simulink model "analog_ext1"  (Simulink 7.6)
settings: Solver=FixedStepDiscrete  StartTime=0.0  StopTime=10.0  FixedStep=1  RelTol=1e-3
libraries: simulink x5
settings Model: Creator=jordan  LastModifiedBy=jordan
settings DataIOCC: LimitDataPoints=off  SaveOutput=off  SignalLogging=off  DSMLogging=off  SaveTime=off
settings OptimizationCC: BlockReduction=off  ConditionallyExecuteInputs=off

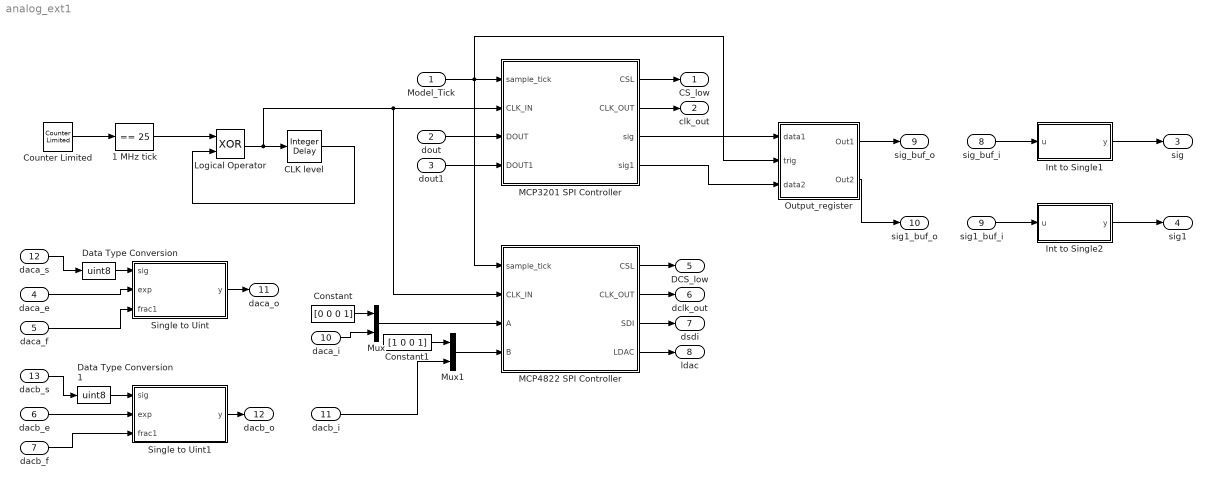
== system analog_ext1 ==
  Model_Tick : Inport  OutDataTypeStr=boolean
  dout : Inport  Port=2  OutDataTypeStr=boolean
  dout1 : Inport  Port=3  OutDataTypeStr=boolean
  daca_e : Inport  Port=4  OutDataTypeStr=uint8
  daca_f : Inport  Port=5  OutDataTypeStr=fixdt(0,24,0)
  dacb_e : Inport  Port=6  OutDataTypeStr=uint8
  dacb_f : Inport  Port=7  OutDataTypeStr=fixdt(0,24,0)
  sig_buf_i : Inport  Port=8  OutDataTypeStr=fixdt(0,12,0)
  sig1_buf_i : Inport  Port=9  OutDataTypeStr=fixdt(0,12,0)
  daca_i : Inport  Port=10  OutDataTypeStr=boolean  PortDimensions=12
  dacb_i : Inport  Port=11  OutDataTypeStr=boolean  PortDimensions=12
  daca_s : Inport  Port=12  OutDataTypeStr=boolean
  dacb_s : Inport  Port=13  OutDataTypeStr=boolean
  1 MHz tick : simulink/Logic and Bit Operations/Compare To Constant  SystemSampleTime=-1  relop===  const=25  LogicOutDataTypeMode=boolean
  CLK level : simulink/Discrete/Integer Delay  NumDelays=1  vinit=0.0  samptime=-1
  Constant : Constant  Value=[0 0 0 1]  OutDataTypeStr=boolean
  Constant1 : Constant  Value=[1 0 0 1]  OutDataTypeStr=boolean
  Counter Limited : simulink/Sources/Counter Limited  SystemSampleTime=-1  uplimit=50  tsamp=-1
  Data Type Conversion : DataTypeConversion  OutDataTypeStr=uint8
  Data Type Conversion1 : DataTypeConversion  OutDataTypeStr=uint8
  Int to Single1 : Stateflow chart  TreatAsAtomicUnit=on
  Int to Single2 : Stateflow chart  TreatAsAtomicUnit=on
  Logical Operator : Logic  Operator=XOR  AllPortsSameDT=off  OutDataTypeStr=boolean
  MCP3201 SPI Controller : Stateflow chart  TreatAsAtomicUnit=on
  MCP4822 SPI Controller : Stateflow chart  TreatAsAtomicUnit=on
  Mux : Mux  Inputs=2
  Mux1 : Mux  Inputs=2
  Output_register : Subsystem
  Single to Uint : Stateflow chart  TreatAsAtomicUnit=on
  Single to Uint1 : Stateflow chart  TreatAsAtomicUnit=on
  CS_low : Outport  OutDataTypeStr=boolean
  clk_out : Outport  Port=2  OutDataTypeStr=boolean
  sig : Outport  Port=3  OutDataTypeStr=uint32  PortDimensions=1
  sig1 : Outport  Port=4  OutDataTypeStr=uint32  PortDimensions=1
  DCS_low : Outport  Port=5  OutDataTypeStr=boolean
  dclk_out : Outport  Port=6  OutDataTypeStr=boolean
  dsdi : Outport  Port=7  OutDataTypeStr=boolean
  ldac : Outport  Port=8  OutDataTypeStr=boolean
  sig_buf_o : Outport  Port=9  OutDataTypeStr=boolean  PortDimensions=12
  sig1_buf_o : Outport  Port=10  OutDataTypeStr=boolean  PortDimensions=12
  daca_o : Outport  Port=11  OutDataTypeStr=fixdt(0,12,0)
  dacb_o : Outport  Port=12  OutDataTypeStr=fixdt(0,12,0)
  wires:
  Counter Limited/1 -> 1 MHz tick/1
  1 MHz tick/1 -> Logical Operator/1
  Logical Operator/1 -> CLK level/1, MCP3201 SPI Controller/2(CLK_IN), MCP4822 SPI Controller/2(CLK_IN)
  CLK level/1 -> Logical Operator/2
  Model_Tick/1 -> MCP3201 SPI Controller/1(sample_tick), MCP4822 SPI Controller/1(sample_tick), Output_register/2(trig)
  MCP3201 SPI Controller/1(CSL) -> CS_low/1
  MCP3201 SPI Controller/2(CLK_OUT) -> clk_out/1
  MCP3201 SPI Controller/3(sig) -> Output_register/1(data1)
  dout/1 -> MCP3201 SPI Controller/3(DOUT)
  MCP3201 SPI Controller/4(sig1) -> Output_register/3(data2)
  dout1/1 -> MCP3201 SPI Controller/4(DOUT1)
  Mux1/1 -> MCP4822 SPI Controller/4(B)
  Constant/1 -> Mux/1
  Mux/1 -> MCP4822 SPI Controller/3(A)
  Constant1/1 -> Mux1/1
  MCP4822 SPI Controller/1(CSL) -> DCS_low/1
  MCP4822 SPI Controller/2(CLK_OUT) -> dclk_out/1
  MCP4822 SPI Controller/3(SDI) -> dsdi/1
  MCP4822 SPI Controller/4(LDAC) -> ldac/1
  Output_register/1(Out1) -> sig_buf_o/1
  Output_register/2(Out2) -> sig1_buf_o/1
  Int to Single1/1(y) -> sig/1
  Int to Single2/1(y) -> sig1/1
  Single to Uint/1(y) -> daca_o/1
  Single to Uint1/1(y) -> dacb_o/1
  daca_s/1 -> Data Type Conversion/1
  daca_e/1 -> Single to Uint/2(exp)
  daca_f/1 -> Single to Uint/3(frac1)
  dacb_e/1 -> Single to Uint1/2(exp)
  dacb_f/1 -> Single to Uint1/3(frac1)
  sig_buf_i/1 -> Int to Single1/1(u)
  sig1_buf_i/1 -> Int to Single2/1(u)
  daca_i/1 -> Mux/2
  dacb_i/1 -> Mux1/2
  dacb_s/1 -> Data Type Conversion1/1
  Data Type Conversion/1 -> Single to Uint/1(sig)
  Data Type Conversion1/1 -> Single to Uint1/1(sig)

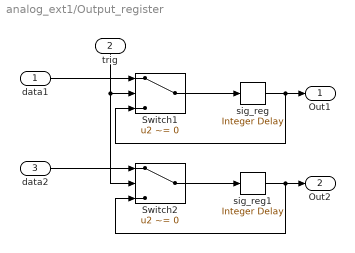
== system analog_ext1/Output_register ==
  data1 : Inport
  trig : Inport  Port=2
  data2 : Inport  Port=3
  Switch1 : Switch  Criteria=u2 ~= 0
  Switch2 : Switch  Criteria=u2 ~= 0
  sig_reg : simulink/Discrete/Integer Delay  NumDelays=1  vinit=0.0  samptime=-1
  sig_reg1 : simulink/Discrete/Integer Delay  NumDelays=1  vinit=0.0  samptime=-1
  Out1 : Outport
  Out2 : Outport  Port=2
  wires:
  Switch1/1 -> sig_reg/1
  sig_reg/1 -> Switch1/3, Out1/1
  Switch2/1 -> sig_reg1/1
  sig_reg1/1 -> Switch2/3, Out2/1
  trig/1 -> Switch2/2, Switch1/2
  data1/1 -> Switch1/1
  data2/1 -> Switch2/1

== stateflow chart MCP3201 SPI Controller ==
  settings: executeAtInitialization=1
  state Wait_Request
  state Get_Sample
  state Wait_CLK_0
  state Get_Sample1
  state Get_Sample2
  state Get_Sample3
  state Receive_Data
  state Receive_Data1
  state Receive_Data2
  state Get_Sample4
  state Get_Sample5
  (default) -> Wait_Request : {CSL=1;
      | CLK_OUT=0;}
  Wait_Request -> Wait_CLK_0 : [sample_tick]
  Wait_CLK_0 -> Get_Sample : [CLK_IN==0]{CSL=0;CLK_OUT=0;}
  Get_Sample -> Get_Sample1 : [CLK_IN]{CLK_OUT=1;}
  Get_Sample1 -> Get_Sample2 : [CLK_IN==0]{CLK_OUT=0;}
  Get_Sample2 -> Get_Sample3 : [CLK_IN]{CLK_OUT=1;}
  Get_Sample3 -> Get_Sample4 : [CLK_IN==0]{CLK_OUT=0;}
  Receive_Data -> (junction 14) : [CLK_IN]{
      | CLK_OUT=1;
      | sig[ind]=DOUT;
      | sig1[ind]=DOUT1;}
  (junction 14) -> (junction 15)
  (junction 15) -> Receive_Data1 [order 2]
  Receive_Data1 -> Receive_Data : [CLK_IN==0]{
      | CLK_OUT=0;
      | ind++;}
  (junction 15) -> Receive_Data2 [order 1] : [ind==11]
  Receive_Data2 -> (junction 16) : [CLK_IN==0]{
      | CLK_OUT=0;
      | CSL=1;}
  (junction 16) -> Wait_Request
  Get_Sample4 -> Get_Sample5 : [CLK_IN]{CLK_OUT=1;}
  Get_Sample5 -> (junction 17) : [CLK_IN==0]{
      | CLK_OUT=0;
      | ind=0;}
  (junction 17) -> Receive_Data
  data: sample_tick input boolean; CSL output boolean; CLK_OUT output boolean; CLK_IN input boolean; DOUT input boolean; sig output boolean size=12; ind local fixdt(0,4,0); sig1 output boolean size=12; DOUT1 input boolean

== stateflow chart MCP4822 SPI Controller ==
  settings: executeAtInitialization=1
  state Wait_Request
  state Wait_CLK
  state Wait_CLK_0
  state DAC_A_Send
  state LatchData
  state Buf_state
  state Buf_state1
  state DAC_A_Send1
  state Wait_CLK1
  state Buf_state2
  (default) -> Wait_Request : {CSL=1;
      | CLK_OUT=0;
      | SDI=0;
      | LDAC=1;}
  Wait_Request -> Wait_CLK_0 : [sample_tick]
  Wait_CLK_0 -> DAC_A_Send : [CLK_IN==0]{
      | CSL=0;
      | CLK_OUT=0;
      | ind=0;
      | SDI=A[0];}
  (junction 56) -> DAC_A_Send
  DAC_A_Send -> Wait_CLK : [CLK_IN]{
      | CLK_OUT=1;
      | ind++;}
  LatchData -> Buf_state2 : [CLK_IN]{
      | LDAC=0;}
  Buf_state2 -> Wait_Request : [CLK_IN==0]{LDAC=1;}
  Wait_CLK -> (junction 57) : [CLK_IN==0]
  (junction 57) -> (junction 56) [order 2] : {CLK_OUT=0;
      | SDI=A[ind];}
  (junction 57) -> Buf_state [order 1] : [ind==16]{CLK_OUT=0;CSL=1;}
  Buf_state -> Buf_state1 : [CLK_IN]
  DAC_A_Send1 -> Wait_CLK1 : [CLK_IN]{
      | CLK_OUT=1;
      | ind++;}
  Wait_CLK1 -> (junction 58) : [CLK_IN==0]
  (junction 58) -> (junction 59) [order 2] : {CLK_OUT=0;
      | SDI=B[ind];}
  (junction 59) -> DAC_A_Send1
  Buf_state1 -> DAC_A_Send1 : [CLK_IN==0]{
      | CSL=0;
      | ind=0;
      | SDI=B[0];}
  (junction 58) -> LatchData [order 1] : [ind==16]{CLK_OUT=0;CSL=1;}
  data: sample_tick input boolean; CSL output boolean; CLK_OUT output boolean; CLK_IN input boolean; A input boolean size=16; ind local fixdt(0,5,0); B input boolean size=16; SDI output boolean; LDAC output boolean

== matlab function Int to Single1 ==
  data: u input fixdt(0,12,0); y output uint32
function y = fcn(u)
%#eml

sig=uint8(0);
exp=uint8(0);
frac=fi(0,0,23,0);

%Transform two's complement integer into unnormalized
%single number
buf=fi(0,0,12,0);
sig=uint8(0);
buf=u;
frac1=fi(buf,0,23,0);

%Normalize floating-point number
buf1=fi(frac1,0,24,0);
p=fi(0,0,5,0);
mask=fi(2^22,0,24,0);
for ind=1:23
    c=bitand(buf1,mask);
    if (c==0)
        buf1=bitshift(buf1,1);
        p=fi(p+1,0,5,0);
    end
end
p=fi(p+1,0,5,0);
buf1=bitshift(fi(frac1,0,24,0),uint8(p));
mask1=fi(2^23-1,0,24,0);
buf1=bitand(buf1,mask1);
frac=fi(buf1,0,23,0);
exp=uint8(127+(22-p));

%Compose floating-point number
z=uint32(0);
if sig
    z=uint32(bitshift(uint32(1),31));
end
buf2=uint32(bitshift(uint32(exp),23));
z=bitor(z,buf2);
z=bitor(z,uint32(frac));
y=z;

== matlab function Int to Single2 ==
  data: u input fixdt(0,12,0); y output uint32
function y = fcn(u)
%#eml

sig=uint8(0);
exp=uint8(0);
frac=fi(0,0,23,0);

%Transform two's complement integer into unnormalized
%single number
buf=fi(0,0,12,0);
sig=uint8(0);
buf=u;
frac1=fi(buf,0,23,0);

%Normalize floating-point number
buf1=fi(frac1,0,24,0);
p=fi(0,0,5,0);
mask=fi(2^22,0,24,0);
for ind=1:23
    c=bitand(buf1,mask);
    if (c==0)
        buf1=bitshift(buf1,1);
        p=fi(p+1,0,5,0);
    end
end
p=fi(p+1,0,5,0);
buf1=bitshift(fi(frac1,0,24,0),uint8(p));
mask1=fi(2^23-1,0,24,0);
buf1=bitand(buf1,mask1);
frac=fi(buf1,0,23,0);
exp=uint8(127+(22-p));

%Compose floating-point number
z=uint32(0);
if sig
    z=uint32(bitshift(uint32(1),31));
end
buf2=uint32(bitshift(uint32(exp),23));
z=bitor(z,buf2);
z=bitor(z,uint32(frac));
y=z;

== matlab function Single to Uint ==
  data: sig input uint8; y output fixdt(0,12,0); exp input uint8; frac1 input fixdt(0,24,0)
function y = fcn(sig, exp, frac1)
%#eml

y=fi(0,0,12,0);
z=int16(0);
if (sig==0)
    if (exp>=127)
        buf=uint32(frac1);
        z=int16(exp)-150;
        y=fi(bitshift(buf,z),0,12,0); %-23+(exp-127)
    end
end

== matlab function Single to Uint1 ==
  data: sig input uint8; y output fixdt(0,12,0); exp input uint8; frac1 input fixdt(0,24,0)
function y = fcn(sig, exp, frac1)
%#eml

y=fi(0,0,12,0);
z=int16(0);
if (sig==0)
    if (exp>=127)
        buf=uint32(frac1);
        z=int16(exp)-150;
        y=fi(bitshift(buf,z),0,12,0); %-23+(exp-127)
    end
end
